simulink model "system_response"  (R2021b)
settings: Solver=VariableStepAuto  StartTime=0.0  StopTime=10  RelTol=1e-3
settings Model: Creator=PARSA  LastModifiedBy=PARSA

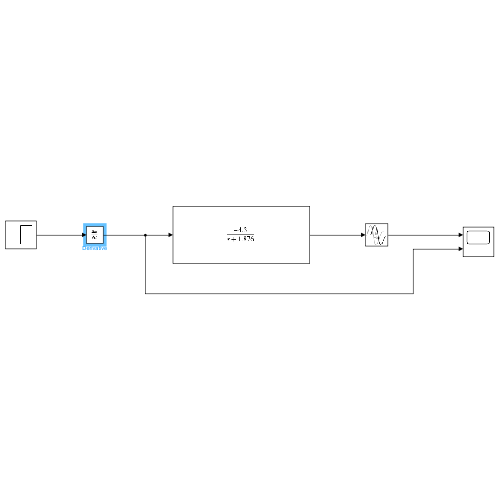
[thumbnail: Simulink's stored preview of the top-level diagram]
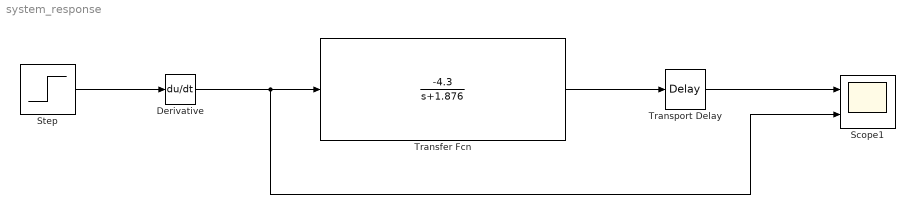
== system system_response ==
  Derivative : Derivative
  Scope1 : Scope  NumInputPorts=2
  Step : Step  SampleTime=0
  Transfer Fcn : TransferFcn  Numerator=[-4.3]  Denominator=[1 1.876]
  Transport Delay : TransportDelay  DelayTime=0.325
  wires:
  Transfer Fcn/1 -> Transport Delay/1
  Transport Delay/1 -> Scope1/1
  Step/1 -> Derivative/1
  Derivative/1 -> Scope1/2, Transfer Fcn/1
